simulink model "bien3310_Design_MJ_f17"  (R2017a)
settings: Solver=ode3  StartTime=0.0  StopTime=20  FixedStep=0.005  RelTol=1e-3  EnableMultiTasking=on
libraries: simulink x3, cstblocks x1
settings Model: Creator=pj  LastModifiedBy=wintersj
settings DataIOCC: LimitDataPoints=on  SaveFormat=StructureWithTime  SignalLoggingSaveFormat=ModelDataLogs
settings OptimizationCC: BlockReduction=off  BufferReuse=off  ExpressionDepthLimit=2147483647  LifeSpan=inf
settings DebuggingCC: AlgebraicLoopMsg=none  UnderspecifiedInitializationDetection=Classic  MergeDetectMultiDrivingBlocksExec=none  MultiTaskRateTransMsg=warning  FcnCallInpInsideContextMsg=warning  UnconnectedInputMsg=none  UnconnectedOutputMsg=none  UnconnectedLineMsg=none  StateNameClashWarn=warning  SFUnexpectedBacktrackingDiag=warning  SFNoUnconditionalDefaultTransitionDiag=warning  SFExecutionAtInitializationDiag=none
settings HardwareCC: ProdBitPerPointer=32  ProdBitPerSizeT=32  ProdBitPerPtrDiffT=32  ProdLargestAtomicFloat=None  ProdIntDivRoundTo=Undefined  ProdEndianess=Unspecified  ProdWordSize=32  ProdHWDeviceType=32-bit Generic
settings ModelReferenceCC: PropagateSignalLabelsOutOfModel=off
settings GRTTargetCC: TargetLangStandard=C89/C90 (ANSI)  GeneratePreprocessorConditionals=Disable all  CombineOutputUpdateFcns=off  GRTInterface=on
settings ConfigComp: CovMetricSettings=dw  CovHtmlReporting=on  CovSaveCumulativeToWorkspaceVar=on  CovSaveSingleToWorkspaceVar=on  CovExternalEMLEnable=off

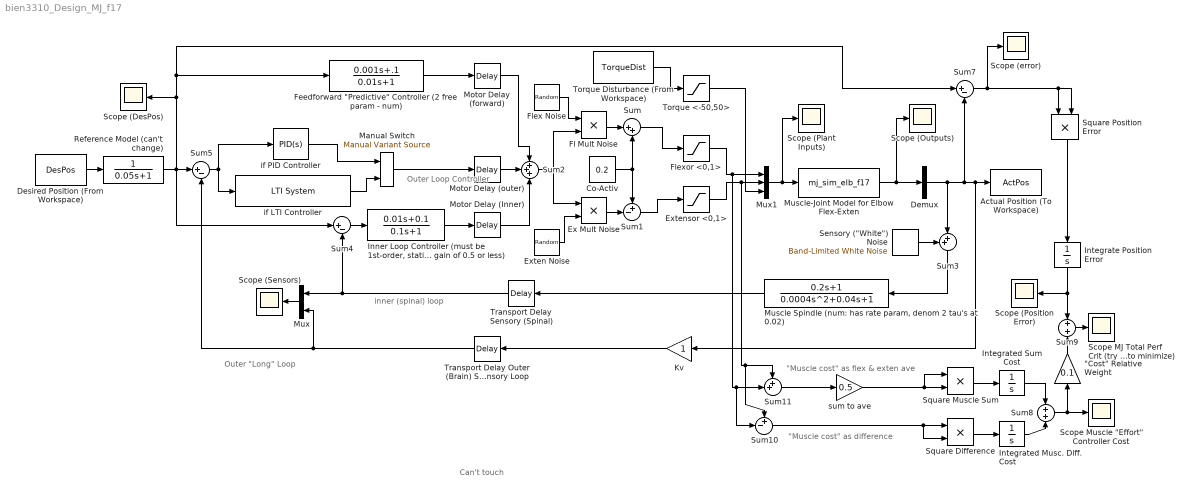
== system bien3310_Design_MJ_f17 ==
  note: Can't touch
  note: Outer Loop
      | Controller
  note: Outer "Long" Loop
  note: inner (spinal) loop
  note: "Muscle cost" as flex & exten ave
  note: "Muscle cost" as difference
  "\"Cost\" Relative Weight" : Gain  Gain=0.1
  Actual Position (To Workspace) : ToWorkspace  VariableName=ActPos  SaveFormat=Structure  SampleTime=-1
  Co-Activ : Constant  Value=0.2
  Demux : Demux  Outputs=3
  Desired Position (From Workspace) : FromWorkspace  VariableName=DesPos  SampleTime=0
  Ex Mult Noise : Product  RndMeth=Zero
  Exten Noise : RandomNumber  Mean=1  Variance=.00000001  SampleTime=0.005
  Extensor <0,1> : Saturate  UpperLimit=1.0  LowerLimit=0
  "Feedforward \"Predictive\" Controller (2 free param - num) " : TransferFcn  Numerator=[0.001 .1]  Denominator=[0.01 1]
  Fl Mult Noise : Product  RndMeth=Zero
  Flex Noise : RandomNumber  Mean=1  Variance=.00000001  Seed=1  SampleTime=0.005
  Flexor <0,1> : Saturate  UpperLimit=1.0  LowerLimit=0
  "Inner Loop Controller (must be 1st-order, static gain of 0.5 or less)" : TransferFcn  Numerator=[0.01 0.1]  Denominator=[0.1 1]
  Integrate Position Error : Integrator
  Integrated Musc. Diff. Cost : Integrator
  Integrated Sum Cost : Integrator
  Kv : Gain
  Manual Switch : simulink/Signal Routing/Manual Variant Source  NumChoices=2  OverrideUsingVariant=V_2
      settings: SourceProductName=Simulink
  Motor Delay (Inner) : TransportDelay  DelayTime=.02
  Motor Delay (forward) : TransportDelay  DelayTime=.04
  Motor Delay (outer) : TransportDelay  DelayTime=.04
  "Muscle Spindle (num: has rate param, denom 2 tau's at 0.02) " : TransferFcn  Numerator=[0.2 1]  Denominator=[0.0004 0.04 1]
  Muscle-Joint Model for Elbow Flex-Exten : S-Function  FunctionName=mj_sim_elb_f17  SFunctionDeploymentMode=off  EnableBusSupport=off
  Mux : Mux  Inputs=2
  Mux1 : Mux  Inputs=3
  Reference Model (can't change) : TransferFcn  Denominator=[0.05 1]
  Scope (DesPos) : Scope
  Scope (Outputs) : Scope
  Scope (Position Error) : Scope
  Scope (Sensors) : Scope
  Scope (error) : Scope
  "Scope Muscle \"Effort\" Controller Cost" : Scope
  Scope (Plant Inputs) : Scope
  Scope MJ Total Perf Crit (try to minimize) : Scope
  "Sensory (\"White\") Noise" : simulink/Sources/Band-Limited White Noise  Cov=[0.0001]  Ts=0.005  seed=[23341]
  Square Difference : Product  RndMeth=Zero
  Square Muscle Sum : Product  RndMeth=Zero
  Square Position Error : Product  RndMeth=Zero
  Sum : Sum  Inputs=|++
  Sum1 : Sum  Inputs=+-|
  Sum10 : Sum  Inputs=+-|
  Sum11 : Sum  Inputs=++|
  Sum2 : Sum  Inputs=+++
  Sum3 : Sum  Inputs=++|
  Sum4 : Sum  Inputs=|+-
  Sum5 : Sum  Inputs=|+-
  Sum7 : Sum  Inputs=|+-
  Sum8 : Sum  Inputs=+|+
  Sum9 : Sum  Inputs=+|+
  Torque <-50,50> : Saturate  UpperLimit=50  LowerLimit=-50
  Torque Disturbance (From Workspace) : FromWorkspace  VariableName=TorqueDist  SampleTime=0
  Transport Delay Outer (Brain) Sensory Loop : TransportDelay  DelayTime=0.05
  Transport Delay Sensory (Spinal) : TransportDelay  DelayTime=0.02
  "if LTI Controller " : cstblocks/LTI System  sys=tf([0.01 0.1 0.1],[0.01 1 0])  IC=[]
  if PID Controller : simulink/Continuous/PID Controller  Controller=PID  TimeDomain=Continuous-time  SampleTime=-1  IntegratorMethod=Forward Euler  FilterMethod=Forward Euler  Form=Parallel  UseFilter=on  ControllerParametersSource=internal  P=0.1  I=0.1  D=0.01  N=100  InitialConditionSource=internal  InitialConditionForIntegrator=0  InitialConditionForFilter=0  ExternalReset=none  LimitOutput=off  UpperSaturationLimit=inf  LowerSaturationLimit=-inf  LinearizeAsGain=on  AntiWindupMode=none  Kb=1  TrackingMode=off  Kt=1  PParamMin=[]  PParamMax=[]  IParamMin=[]  IParamMax=[]  DParamMin=[]  DParamMax=[]  NParamMin=[]  NParamMax=[]  KbParamMin=[]  KbParamMax=[]  KtParamMin=[]  KtParamMax=[]  POutMin=[]  POutMax=[]  IOutMin=[]  IOutMax=[]  DOutMin=[]  DOutMax=[]  NOutMin=[]  NOutMax=[]  KbOutMin=[]  KbOutMax=[]  KtOutMin=[]  KtOutMax=[]  IntegratorOutMin=[]  IntegratorOutMax=[]  FilterOutMin=[]  FilterOutMax=[]  SumOutMin=[]  SumOutMax=[]  SumI1OutMin=[]  SumI1OutMax=[]  SumI2OutMin=[]  SumI2OutMax=[]  SumI3OutMin=[]  SumI3OutMax=[]  SumDOutMin=[]  SumDOutMax=[]  SaturationOutMin=[]  SaturationOutMax=[]  IntegratorContinuousStateAttributes=''  IntegratorStateMustResolveToSignalObject=off  IntegratorRTWStateStorageClass=Auto  FilterContinuousStateAttributes=''  FilterStateMustResolveToSignalObject=off  FilterRTWStateStorageClass=Auto  DifferentiatorICPrevScaledInput=0  DifferentiatorOutMin=[]  DifferentiatorOutMax=[]  InitialConditionSetting=State (most efficient)
  sum to ave : Gain  Gain=0.5
  wires:
  Mux1/1 -> Muscle-Joint Model for Elbow Flex-Exten/1, Scope (Plant Inputs)/1
  Muscle-Joint Model for Elbow Flex-Exten/1 -> Scope (Outputs)/1, Demux/1
  Co-Activ/1 -> Sum/2, Sum1/1
  Sum/1 -> Flexor <0,1>/1
  Sum1/1 -> Extensor <0,1>/1
  Torque Disturbance (From Workspace)/1 -> Torque <-50,50>/1
  "Sensory (\"White\") Noise"/1 -> Sum3/1
  Sum3/1 -> "Muscle Spindle (num: has rate param, denom 2 tau's at 0.02) "/1
  Demux/2 -> Sum7/2, Kv/1, Actual Position (To Workspace)/1, Sum3/2
  Transport Delay Sensory (Spinal)/1 -> Mux/1, Sum4/2
  Fl Mult Noise/1 -> Sum/1
  Ex Mult Noise/1 -> Sum1/2
  Flex Noise/1 -> Fl Mult Noise/1
  Exten Noise/1 -> Ex Mult Noise/2
  Sum5/1 -> if PID Controller/1, "if LTI Controller "/1
  Transport Delay Outer (Brain) Sensory Loop/1 -> Mux/2, Sum5/2
  Mux/1 -> Scope (Sensors)/1
  Extensor <0,1>/1 -> Sum10/1, Sum11/1, Mux1/2
  Torque <-50,50>/1 -> Mux1/3
  Sum7/1 -> Square Position Error/2, Square Position Error/1, Scope (error)/1
  Square Position Error/1 -> Integrate Position Error/1
  Integrate Position Error/1 -> Sum9/1, Scope (Position Error)/1
  Kv/1 -> Transport Delay Outer (Brain) Sensory Loop/1
  Flexor <0,1>/1 -> Mux1/1, Sum10/2, Sum11/2
  Sum2/1 -> Ex Mult Noise/1, Fl Mult Noise/2
  Square Muscle Sum/1 -> Integrated Sum Cost/1
  Sum9/1 -> Scope MJ Total Perf Crit (try to minimize)/1
  "\"Cost\" Relative Weight"/1 -> Sum9/2
  Square Difference/1 -> Integrated Musc. Diff. Cost/1
  Integrated Sum Cost/1 -> Sum8/1
  Integrated Musc. Diff. Cost/1 -> Sum8/2
  Sum8/1 -> "Scope Muscle \"Effort\" Controller Cost"/1, "\"Cost\" Relative Weight"/1
  "Inner Loop Controller (must be 1st-order, static gain of 0.5 or less)"/1 -> Motor Delay (Inner)/1
  Sum4/1 -> "Inner Loop Controller (must be 1st-order, static gain of 0.5 or less)"/1
  "Muscle Spindle (num: has rate param, denom 2 tau's at 0.02) "/1 -> Transport Delay Sensory (Spinal)/1
  Motor Delay (Inner)/1 -> Sum2/3
  Motor Delay (outer)/1 -> Sum2/2
  Desired Position (From Workspace)/1 -> Reference Model (can't change)/1
  Reference Model (can't change)/1 -> Sum4/1, Sum7/1, "Feedforward \"Predictive\" Controller (2 free param - num) "/1, Scope (DesPos)/1, Sum5/1
  Motor Delay (forward)/1 -> Sum2/1
  "Feedforward \"Predictive\" Controller (2 free param - num) "/1 -> Motor Delay (forward)/1
  Sum10/1 -> Square Difference/1, Square Difference/2
  Sum11/1 -> sum to ave/1
  Manual Switch/1 -> Motor Delay (outer)/1
  "if LTI Controller "/1 -> Manual Switch/2
  if PID Controller/1 -> Manual Switch/1
  sum to ave/1 -> Square Muscle Sum/1, Square Muscle Sum/2
